simulink model "RadBtwPlatesEx"  (R2015a)
settings: Solver=FixedStepDiscrete  StartTime=0.0  StopTime=tsim  FixedStep=dt  RelTol=1e-3
values from neighbouring files (symbols this model uses):
  Cp = 6.92*ones(length(x1),1)'    [run_RadBtwPlates.m]
  eps_earth = 0.5    [run_RadBtwPlates.m]
  eps_space = 1    [run_RadBtwPlates.m]
  k = 0.0328*ones(length(x1),1)'    [run_RadBtwPlates.m]
  rho = 5.238864896*ones(length(x1),1)'    [run_RadBtwPlates.m]
  To1 = 500*ones(length(x1),1)'    [run_RadBtwPlates.m]
  To2 = 500*ones(length(x2),1)'    [run_RadBtwPlates.m]
  Tsink_earth = 464.4    [run_RadBtwPlates.m]
  Tsink_space = 4.9    [run_RadBtwPlates.m]
  x1 = linspace(0,0.25/12,20)    [run_RadBtwPlates.m]
  x2 = x1    [run_RadBtwPlates.m]
libraries: lib_Conduction_HeatX1DVarPropsAndGenBCs x2, lib_Radiation_HeatXCoeffNonRefSink x2, lib_Radiation_HeatXCoeffRefPlanar x1
settings Model: Creator=jlkratz  LastModifiedBy=jlkratz

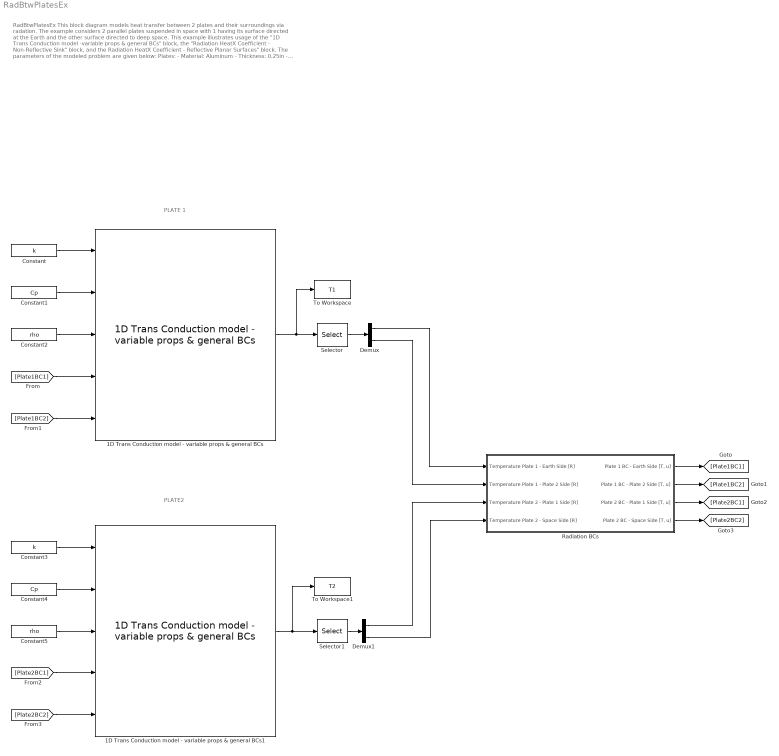
== system RadBtwPlatesEx ==
  note: PLATE 1
  note: RadBtwPlatesEx
      |
      | This block diagram models heat transfer between 2 plates and their surroundings via radation. The example
      | considers 2 parallel plates suspended in space with 1 having its surface directed at the Earth and the other surface
      | directed to deep space. This example illustrates usage of the "1D Trans Conduction model -variable props & general
      | BCs" block, the "Radiation HeatX Coefficient - Non-Reflective Sink" block, and the Radiation HeatX Coefficient -
      | Reflective Planar Surfaces" block. The parameters of the modeled problem are given below:
      | Plates:
      | - Material: Aluminum
      | - Thickness: 0.25in
      | - Emissivity: 1 (treated and painted black to modify emissivity)
      | - Initial Temperature: 500R throughout
      | Radiation with Earth:
      | - Emissivity: 0.5
      | - Sink Temperature: 464R
      | Radiation with Space:
      | - Emissivity: 1
      | - Sink Temperature: 4.9R
  note: PLATE2
  1D Trans Conduction model - variable props & general BCs : lib_Conduction_HeatX1DVarPropsAndGenBCs/1D Trans Conduction model - variable props & general BCs  x_M=x1  T0_M=To1  dt_M=dt  a_M=off  convin_M=off  radin_M=on  condin_M=off  convout_M=off  radout_M=on  condout_M=off  BN_M=double(gcb)
  1D Trans Conduction model - variable props & general BCs1 : lib_Conduction_HeatX1DVarPropsAndGenBCs/1D Trans Conduction model - variable props & general BCs  x_M=x2  T0_M=To2  dt_M=dt  a_M=off  convin_M=off  radin_M=on  condin_M=off  convout_M=off  radout_M=on  condout_M=off  BN_M=double(gcb)
  Constant : Constant  Value=k
  Constant1 : Constant  Value=Cp
  Constant2 : Constant  Value=rho
  Constant3 : Constant  Value=k
  Constant4 : Constant  Value=Cp
  Constant5 : Constant  Value=rho
  Demux : Demux  Outputs=2
  Demux1 : Demux  Outputs=2
  Radiation BCs : Subsystem
  Selector : Selector  InputPortWidth=length(x1)  Indices=[1 length(x1)]
  Selector1 : Selector  InputPortWidth=length(x2)  Indices=[1 length(x2)]
  To Workspace : ToWorkspace  VariableName=T1  SaveFormat=Timeseries  SampleTime=-1
  To Workspace1 : ToWorkspace  VariableName=T2  SaveFormat=Timeseries  SampleTime=-1
  wires:
  Constant/1 -> 1D Trans Conduction model - variable props & general BCs/1
  Constant1/1 -> 1D Trans Conduction model - variable props & general BCs/2
  Constant2/1 -> 1D Trans Conduction model - variable props & general BCs/3
  [Plate1BC1] -> 1D Trans Conduction model - variable props & general BCs/4
  1D Trans Conduction model - variable props & general BCs/1 -> To Workspace/1, Selector/1
  [Plate1BC2] -> 1D Trans Conduction model - variable props & general BCs/5
  Selector/1 -> Demux/1
  1D Trans Conduction model - variable props & general BCs1/1 -> To Workspace1/1, Selector1/1
  Selector1/1 -> Demux1/1
  Demux/1 -> Radiation BCs/1(Temperature Plate 1 - Earth Side [R])
  Demux/2 -> Radiation BCs/2(Temperature Plate 1 - Plate 2 Side [R])
  Demux1/1 -> Radiation BCs/3(Temperature Plate 2 - Plate 1 Side [R])
  Demux1/2 -> Radiation BCs/4(Temperature Plate 2 - Space Side [R])
  Constant3/1 -> 1D Trans Conduction model - variable props & general BCs1/1
  Constant4/1 -> 1D Trans Conduction model - variable props & general BCs1/2
  Constant5/1 -> 1D Trans Conduction model - variable props & general BCs1/3
  Radiation BCs/1("Plate 1 BC - Earth Side [T, u]") -> [Plate1BC1]
  Radiation BCs/2("Plate 1 BC - Plate 2 Side [T, u]") -> [Plate1BC2]
  Radiation BCs/3("Plate 2 BC - Plate 1 Side [T, u]") -> [Plate2BC1]
  Radiation BCs/4("Plate 2 BC - Space Side [T, u]") -> [Plate2BC2]
  [Plate2BC2] -> 1D Trans Conduction model - variable props & general BCs1/5
  [Plate2BC1] -> 1D Trans Conduction model - variable props & general BCs1/4

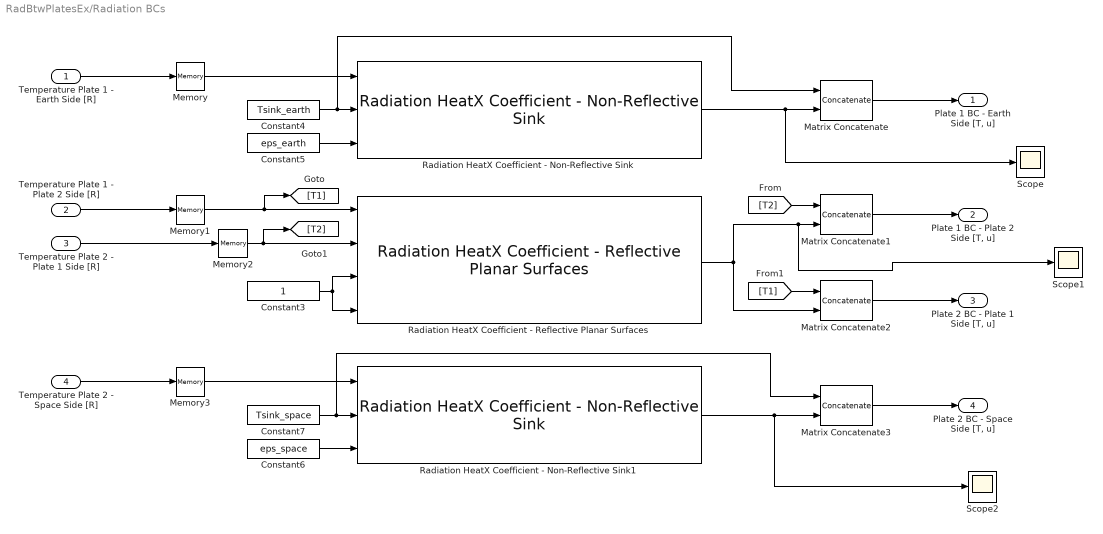
== system RadBtwPlatesEx/Radiation BCs ==
  Temperature Plate 1 - Earth Side [R] : Inport
  Temperature Plate 1 - Plate 2 Side [R] : Inport  Port=2
  Temperature Plate 2 - Plate 1 Side [R] : Inport  Port=3
  Temperature Plate 2 - Space Side [R] : Inport  Port=4
  Constant3 : Constant
  Constant4 : Constant  Value=Tsink_earth
  Constant5 : Constant  Value=eps_earth
  Constant6 : Constant  Value=eps_space
  Constant7 : Constant  Value=Tsink_space
  Matrix Concatenate{,1..3} (4 alike) : Concatenate  ConcatenateDimension=2
  Memory : Memory  X0=To1(1)
  Memory1 : Memory  X0=To1(end)
  Memory2 : Memory  X0=To2(1)
  Memory3 : Memory  X0=To2(end)
  Radiation HeatX Coefficient - Non-Reflective Sink : lib_Radiation_HeatXCoeffNonRefSink/Radiation HeatX Coefficient - Non-Reflective Sink
  Radiation HeatX Coefficient - Non-Reflective Sink1 : lib_Radiation_HeatXCoeffNonRefSink/Radiation HeatX Coefficient - Non-Reflective Sink
  Radiation HeatX Coefficient - Reflective Planar Surfaces : lib_Radiation_HeatXCoeffRefPlanar/Radiation HeatX Coefficient - Reflective Planar Surfaces
  Scope : Scope
  Scope1 : Scope
  Scope2 : Scope
      settings: SaveName=ScopeData2
  "Plate 1 BC - Earth Side [T, u]" : Outport
  "Plate 1 BC - Plate 2 Side [T, u]" : Outport  Port=2
  "Plate 2 BC - Plate 1 Side [T, u]" : Outport  Port=3
  "Plate 2 BC - Space Side [T, u]" : Outport  Port=4
  wires:
  Temperature Plate 1 - Plate 2 Side [R]/1 -> Memory1/1
  Temperature Plate 1 - Earth Side [R]/1 -> Memory/1
  Constant5/1 -> Radiation HeatX Coefficient - Non-Reflective Sink/3
  Constant3/1 -> Radiation HeatX Coefficient - Reflective Planar Surfaces/3, Radiation HeatX Coefficient - Reflective Planar Surfaces/4
  Constant4/1 -> Matrix Concatenate/1, Radiation HeatX Coefficient - Non-Reflective Sink/2
  Temperature Plate 2 - Plate 1 Side [R]/1 -> Memory2/1
  Temperature Plate 2 - Space Side [R]/1 -> Memory3/1
  Constant6/1 -> Radiation HeatX Coefficient - Non-Reflective Sink1/3
  Constant7/1 -> Matrix Concatenate3/1, Radiation HeatX Coefficient - Non-Reflective Sink1/2
  Radiation HeatX Coefficient - Non-Reflective Sink/1 -> Scope/1, Matrix Concatenate/2
  [T2] -> Matrix Concatenate1/1
  [T1] -> Matrix Concatenate2/1
  Matrix Concatenate/1 -> "Plate 1 BC - Earth Side [T, u]"/1
  Matrix Concatenate1/1 -> "Plate 1 BC - Plate 2 Side [T, u]"/1
  Matrix Concatenate2/1 -> "Plate 2 BC - Plate 1 Side [T, u]"/1
  Radiation HeatX Coefficient - Non-Reflective Sink1/1 -> Scope2/1, Matrix Concatenate3/2
  Matrix Concatenate3/1 -> "Plate 2 BC - Space Side [T, u]"/1
  Memory/1 -> Radiation HeatX Coefficient - Non-Reflective Sink/1
  Memory1/1 -> [T1], Radiation HeatX Coefficient - Reflective Planar Surfaces/1
  Memory2/1 -> [T2], Radiation HeatX Coefficient - Reflective Planar Surfaces/2
  Memory3/1 -> Radiation HeatX Coefficient - Non-Reflective Sink1/1
  Radiation HeatX Coefficient - Reflective Planar Surfaces/1 -> Matrix Concatenate1/2, Scope1/1, Matrix Concatenate2/2
